simulink model "Inverted_pendulum"  (R2023a)
settings: Solver=ode4  StartTime=0.0  StopTime=inf  FixedStep=0.002  RelTol=1e-3  EnableMultiTasking=on
PostLoadFcn:
  | qc_set_target_type(getConfigSet(bdroot, 'QUARC Default Target Configuration'));
values from neighbouring files (symbols this model uses):
  a = Jeq+m*r^2+zeta_g*Kg^2*Jm    (= 0.011068995)    [LQR.m]    (also in LQRtune.m; SS_Model.m)
  A = [0 0 1 0; 0 0 0 1; MiG MiD]    [LQR.m]    (also in LQRtune.m; SS_Model.m)
  b = m*L*r    (= 0.0045015625)    [LQR.m]    (also in LQRtune.m; SS_Model.m)
  B = [0; 0; MiB]    [LQR.m]    (also in LQRtune.m; SS_Model.m)
  c = 4/3*m*L^2    (= 0.00467604166667)    [LQR.m]    (also in LQRtune.m; SS_Model.m)
  C = eye(4)    [LQR.m]    (also in LQRtune.m; SS_Model.m)
  d = m*g*L    (= 0.205396875)    [LQR.m]    (also in LQRtune.m; SS_Model.m)
  D = [0 0 0 0]'    [LQR.m]    (also in LQRtune.m; SS_Model.m)
  f = (zeta_m*zeta_g*Kt*Kg)/Rm    (= 0.1282365)    [LQR.m]    (also in LQRtune.m; SS_Model.m)
  Ts = .002    (= 0.002)    [LQR.m]    (also in LQRtune.m; SS_Model.m)
  w1 = 10*w0    (= 54.9778714378)    [LQR.m]    (also in LQRtune.m = 250; SS_Model.m)
undefined symbols (not defined in the file or in its folder): HIL
libraries: quarc_library x5
settings Model: SimulationMode=external  ExtModeTrigDuration=10000  Creator=MLevis  LastModifiedBy=quarc_user
settings SolverCC: AlgebraicLoopSolver=TrustRegion  PositivePriorityOrder=on  AutoInsertRateTranBlk=on
settings DataIOCC: LimitDataPoints=on  SaveFormat=Array  SignalLoggingSaveFormat=ModelDataLogs  ReturnWorkspaceOutputs=off
settings OptimizationCC: ExpressionDepthLimit=2147483647  InitFltsAndDblsToZero=on
settings DebuggingCC: SaveWithParameterizedLinksMsg=none  UnderspecifiedInitializationDetection=Classic  MergeDetectMultiDrivingBlocksExec=none  SolverPrmCheckMsg=warning  MultiTaskDSMMsg=warning  MultiTaskCondExecSysMsg=none  FcnCallInpInsideContextMsg=warning  UnconnectedInputMsg=warning  UnconnectedOutputMsg=warning  UnconnectedLineMsg=warning  StateNameClashWarn=warning  SFUnexpectedBacktrackingDiag=warning  SFNoUnconditionalDefaultTransitionDiag=warning  SFExecutionAtInitializationDiag=none  ArithmeticOperatorsInVariantConditions=warning
settings ModelReferenceCC: EnableRefExpFcnMdlSchedulingChecks=on  PropagateSignalLabelsOutOfModel=off
settings SFSimCC: SimUseLocalCustomCode=off  CustomCodeUndefinedFunction=UseInterfaceOnly
settings RTWCC: Description=QUARC Win64 Target Using Toolchain  SystemTargetFile=quarc_win64.tlc  TemplateMakefile=quarc_default_tmf  RTWUseLocalCustomCode=off  Toolchain=QUARC win64 | nmake (64-bit Windows)  BuildConfiguration=Faster Runs  DLArmComputeVersion=19.05
settings CodeAppCC: StateflowObjectComments=on
settings STFCustomTargetCC: TargetLangStandard=C89/C90 (ANSI)  SystemTargetFile=quarc_win64.tlc
settings GRTTargetCC: TargetLangStandard=C89/C90 (ANSI)  ParMdlRefBuildCompliant=off  CompOptLevelCompliant=off  CombineOutputUpdateFcns=off  MatFileLogging=off  CPPClassGenCompliant=off  GRTInterface=on  ExtMode=on  ExtModeMexFile=quarc_comm
settings ConfigComp: CovMetricSettings=dw  CovSaveCumulativeToWorkspaceVar=on  CovSaveSingleToWorkspaceVar=on  CovExternalEMLEnable=off

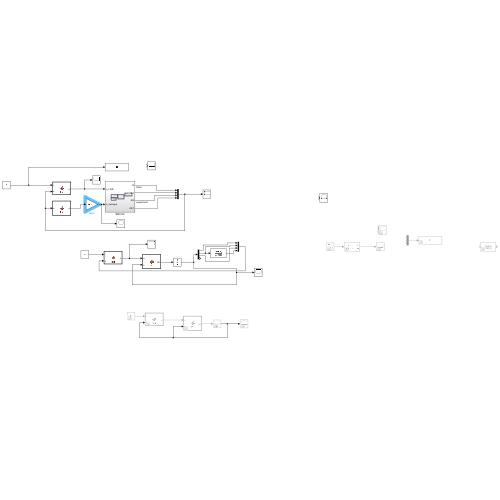
[thumbnail: Simulink's stored preview of the top-level diagram]
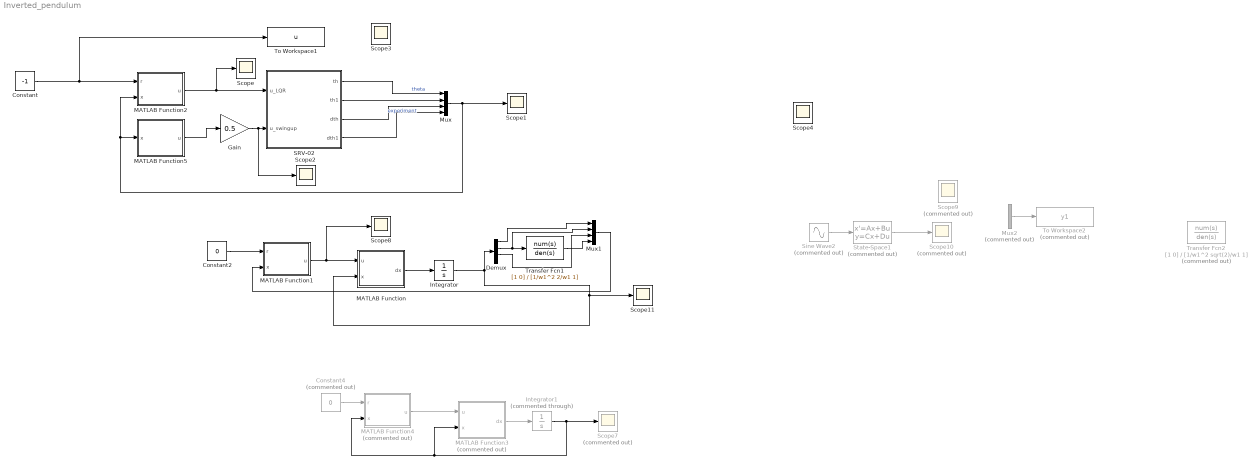
== system Inverted_pendulum ==
  Constant : Constant  Value=-1
  Constant2 : Constant  Value=0
  Constant4 : Constant  Commented=on  Value=0
  Demux : Demux
  Gain : Gain  Gain=0.5
  Integrator : Integrator  InitialCondition=[0; deg2rad(5); 0; 0]
  Integrator1 : Integrator  Commented=through  InitialCondition=[0; deg2rad(.1); 0; 0]
  MATLAB Function : MATLAB Function  TreatAsAtomicUnit=on
  MATLAB Function1 : MATLAB Function  TreatAsAtomicUnit=on
  MATLAB Function2 : MATLAB Function  TreatAsAtomicUnit=on
  MATLAB Function3 : MATLAB Function  Commented=on  TreatAsAtomicUnit=on
  MATLAB Function4 : MATLAB Function  Commented=on  TreatAsAtomicUnit=on
  MATLAB Function5 : MATLAB Function  TreatAsAtomicUnit=on
  Mux : Mux
  Mux1 : Mux
  Mux2 : Mux  Commented=on
  SRV-02 : Subsystem
  Scope{,1..4,8,11} (7 alike) : Scope
  Scope10 : Scope  Commented=on
  Scope7 : Scope  Commented=on
  Scope9 : Scope  Commented=on  NumInputPorts=3
  Sine Wave2 : Sin  Commented=on  SampleTime=0
  State-Space1 : StateSpace  Commented=on  A=A  B=B  C=C  D=D  InitialCondition=0
  To Workspace1 : ToWorkspace  VariableName=u  SampleTime=Ts
  To Workspace2 : ToWorkspace  Commented=on  VariableName=y1  SampleTime=Ts
  Transfer Fcn1 : TransferFcn  Numerator=[1 0]  Denominator=[1/w1^2 2/w1 1]
  Transfer Fcn2 : TransferFcn  Commented=on  Numerator=[1 0]  Denominator=[1/w1^2 sqrt(2)/w1 1]
  wires:
  SRV-02/1(th) -> Mux/1  "theta"
  SRV-02/3(dth) -> Mux/3  "experiment"
  SRV-02/4(dth1) -> Mux/4
  Constant/1 -> MATLAB Function2/1(r), To Workspace1/1
  SRV-02/2(th1) -> Mux/2
  Integrator/1 -> Scope11/1, MATLAB Function/2(x), Demux/1
  MATLAB Function1/1(u) -> Scope8/1, MATLAB Function/1(u)
  Constant4/1 -> MATLAB Function4/1(r)
  MATLAB Function4/1(u) -> MATLAB Function3/1(u)
  Integrator1/1 -> Scope7/1, MATLAB Function3/2(x), MATLAB Function4/2(x)
  MATLAB Function3/1(dx) -> Integrator1/1
  MATLAB Function/1(dx) -> Integrator/1
  Demux/2 -> Mux1/2, Transfer Fcn1/1
  Demux/1 -> Mux1/1
  Mux1/1 -> MATLAB Function1/2(x)
  Demux/3 -> Mux1/3
  Transfer Fcn1/1 -> Mux1/4
  Sine Wave2/1 -> State-Space1/1
  State-Space1/1 -> Scope10/1
  Mux2/1 -> To Workspace2/1
  Constant2/1 -> MATLAB Function1/1(r)
  Mux/1 -> Scope1/1, MATLAB Function2/2(x), MATLAB Function5/1(x)
  MATLAB Function2/1(u) -> Scope/1, SRV-02/1(u_LQR)
  MATLAB Function5/1(u) -> Gain/1
  Gain/1 -> Scope2/1, SRV-02/2(u_swingup)

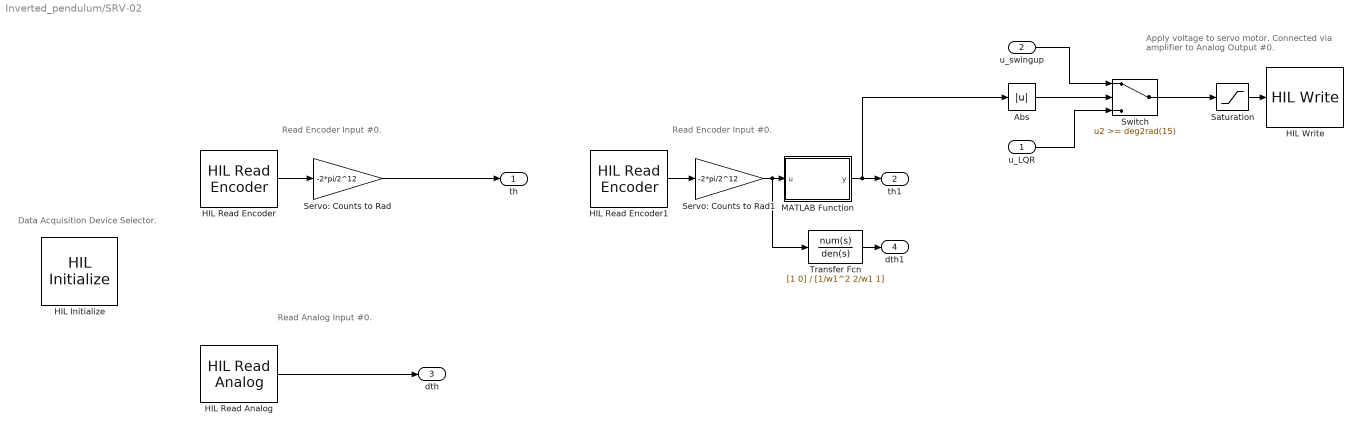
== system Inverted_pendulum/SRV-02 ==
  note: Apply voltage to servo motor.
      | Connected via amplifier to Analog Output #0.
  note: Read Analog Input #0.
  note: Read Encoder Input #0.
  note: Data Acquisition Device Selector.
  note: Read Encoder Input #0.
  u_LQR : Inport
  u_swingup : Inport  Port=2
  Abs : Abs  SaturateOnIntegerOverflow=off
  HIL Initialize : quarc_library/Data Acquisition/Generic/Configuration/HIL Initialize  object_name=HIL-1  board_type=q2_usb  board_number=0  board_options=d0=digital;d1=digital;led=auto;update_rate=normal;decimation=1  exclusive=off  active=off  hardware_clocks=[0]  clock_modes=[]  initial_clock_frequencies=[]  set_clock_params_at_start=off  set_clock_params_at_switch_in=off  set_clock_frequencies_at_start=off  set_clock_frequencies_at_switch_in=off  analog_input_channels=[0:1]  analog_input_configurations=[]  analog_input_maximums=10  analog_input_minimums=-10  set_analog_input_params_at_start=on  set_analog_input_params_at_switch_in=off  analog_output_channels=[0:1]  analog_output_maximums=10  analog_output_minimums=-10  initial_analog_outputs=[0]  final_analog_outputs=[0]  watchdog_analog_outputs=0  set_analog_output_params_at_start=on  set_analog_output_params_at_switch_in=off  set_analog_outputs_at_start=on  set_analog_outputs_at_switch_in=off  set_analog_outputs_at_terminate=on  set_analog_outputs_at_switch_out=off  set_analog_outputs_on_watchdog=off  digital_input_channels=[]  digital_output_channels=[]  digital_output_configuration=[]  initial_digital_outputs=[1]  final_digital_outputs=[1]  watchdog_digital_outputs=[1]  set_digital_output_params_at_start=off  set_digital_output_params_at_switch_in=off  set_digital_outputs_at_start=on  set_digital_outputs_at_switch_in=off  set_digital_outputs_at_terminate=on  set_digital_outputs_at_switch_out=off  set_digital_outputs_on_watchdog=off  encoder_channels=[0:1]  quadrature=[4]  encoder_filter_frequency=[]  initial_encoder_counts=[0]  set_encoder_params_at_start=on  set_encoder_params_at_switch_in=off  set_encoder_counts_at_start=on  set_encoder_counts_at_switch_in=off  pwm_channels=[]  pwm_modes=[0]  pwm_frequency=1/0.020  pwm_configuration=[]  pwm_alignment=[]  pwm_polarity=[]  pwm_leading_deadband=[]  pwm_trailing_deadband=[]  initial_pwm_outputs=[0]  final_pwm_outputs=[0]  watchdog_pwm_outputs=[0]  set_pwm_params_at_start=on  set_pwm_params_at_switch_in=off  set_pwm_outputs_at_start=on  set_pwm_outputs_at_switch_in=off  set_pwm_outputs_at_terminate=on  set_pwm_outputs_at_switch_out=off  set_pwm_outputs_on_watchdog=off  other_output_channels=[]  initial_other_outputs=[]  final_other_outputs=[]  watchdog_other_outputs=[]  set_other_outputs_at_start=off  set_other_outputs_at_switch_in=off  set_other_outputs_at_terminate=off  set_other_outputs_at_switch_out=off  set_other_outputs_on_watchdog=off
  HIL Read Analog : quarc_library/Data Acquisition/Generic/Immediate I//O/HIL Read Analog  object_name=HIL-1  channels=[0]  sample_time=qc_get_step_size  active=on  vector_output=off
  HIL Read Encoder : quarc_library/Data Acquisition/Generic/Immediate I//O/HIL Read Encoder  object_name=HIL-1  channels=0  sample_time=qc_get_step_size  active=on  vector_output=off  data_type_mode=Inherit via back propagation  data_type=double
  HIL Read Encoder1 : quarc_library/Data Acquisition/Generic/Immediate I//O/HIL Read Encoder  object_name=HIL-1  channels=1  sample_time=qc_get_step_size  active=on  vector_output=off  data_type_mode=Inherit via back propagation  data_type=double
  HIL Write : quarc_library/Data Acquisition/Generic/Immediate I//O/HIL Write  Tag=unassigned  object_name=HIL-1  analog_channels=0  pwm_channels=[]  digital_channels=[]  other_channels=[]  sample_time=-1  active=off  vector_input=off
  MATLAB Function : MATLAB Function  TreatAsAtomicUnit=on
  Saturation : Saturate  UpperLimit=10  LowerLimit=-10
  Servo: Counts to Rad : Gain  Gain=-2*pi/2^12
  Servo: Counts to Rad1 : Gain  Gain=-2*pi/2^12
  Switch : Switch  Threshold=deg2rad(15)  SaturateOnIntegerOverflow=off  InputSameDT=off
  Transfer Fcn : TransferFcn  Numerator=[1 0]  Denominator=[1/w1^2 2/w1 1]
  th : Outport
  th1 : Outport  Port=2
  dth : Outport  Port=3
  dth1 : Outport  Port=4
  wires:
  HIL Read Encoder/1 -> Servo: Counts to Rad/1
  Saturation/1 -> HIL Write/1
  HIL Read Analog/1 -> dth/1
  HIL Read Encoder1/1 -> Servo: Counts to Rad1/1
  Servo: Counts to Rad1/1 -> Transfer Fcn/1, MATLAB Function/1(u)
  Transfer Fcn/1 -> dth1/1
  Switch/1 -> Saturation/1
  MATLAB Function/1(y) -> Abs/1, th1/1
  Abs/1 -> Switch/2
  u_swingup/1 -> Switch/1
  u_LQR/1 -> Switch/3
  Servo: Counts to Rad/1 -> th/1

== matlab function Inverted_pendulum/MATLAB Function ==
  data: u input; dx output; x input; a parameter; b parameter; c parameter; d parameter; e parameter; f parameter
function dx = fcn(u,x,a, b, c, d, e, f)

Ma = [a -b*cos(x(2))
    -b*cos(x(2)) c];


dx = zeros(4,1);
dx(1:2,:) = x(3:4);
Co = [0 -b*sin(x(2))*x(4); 0 0];
Go = [0; d*sin(x(2))];
Do = [e 0; 0 0];
Bo = [f; 0];
Eq = Co*[x(3); x(4)] + Go - Do*[x(3);x(4)] + Bo*u;
dx(3:4,:) = Ma\[Eq];

== matlab function Inverted_pendulum/SRV-02/MATLAB Function ==
  data: u input; y output
function y = fcn(u)

y = mod(u,2*pi)-pi;

== matlab function Inverted_pendulum/MATLAB Function1 ==
  data: r input; u output; x input; K parameter
function u = fcn(r,x,K)

u = -K*x;

== matlab function Inverted_pendulum/MATLAB Function2 ==
  data: r input; u output; x input; K parameter
function u = fcn(r,x,K)

u = -K*x;

== matlab function Inverted_pendulum/MATLAB Function3 ==
  data: u input; dx output; x input; a parameter; b parameter; c parameter; d parameter; e parameter; f parameter
function dx = fcn(u,x,a, b, c, d, e, f)

Ma = [a -b
     -b c];


dx = zeros(4,1);
dx(1:2,:) = x(3:4);
Go = [0; d*x(2)];
Do = [e 0; 0 0];
Bo = [f; 0];
Eq = Go - Do*[x(3);x(4)] + Bo*u;
dx(3:4,:) = Ma\[Eq];

== matlab function Inverted_pendulum/MATLAB Function4 ==
  data: r input; u output; x input; K parameter
function u = fcn(r,x,K)

u = -K*x;

== matlab function Inverted_pendulum/MATLAB Function5 ==
  data: u output; x input; d parameter; c parameter
function u  = fcn(x,d, c)
if abs(x(2)) ~= pi && x(4) ~= 0
    E = d*cos(x(2)) + 0.5*c*x(4)^2;
    Etarget = 2*d;

    if E<Etarget
        u = cos(x(2))*x(4);
    else
        u = 0;
    end
else
    u = 4/.2;
end
